simulink model "sim_sil_target_PWM_s32k1xx"  (Simulink 9.0)
settings: Solver=FixedStepDiscrete  StartTime=0.0  StopTime=12  FixedStep=1  RelTol=1e-3  EnableMultiTasking=on
InitFcn:
  | mbd_s32k_consistency_checks(bdroot(gcs));
undefined symbols (not defined in the file): LQFP
libraries: mbd_s32k1xx_ec_toolbox x2
settings Model: Creator=NXP MBDT Team  LastModifiedBy=nxf35172
settings DataIOCC: ExternalInput=off  InitialState=off  LimitDataPoints=on  SaveOutput=off  SignalLogging=off  SaveTime=off
settings OptimizationCC: DefaultParameterBehavior=Inlined  EnhancedBackFolding=on  PassReuseOutputArgsAs=Individual arguments  LifeSpan=auto  OptimizeBlockOrder=speed  DifferentSizesBufferReuse=on
settings DebuggingCC: UnderspecifiedInitializationDetection=Simplified  MergeDetectMultiDrivingBlocksExec=error  SolverPrmCheckMsg=warning  InheritedTsInSrcMsg=none  SingleTaskRateTransMsg=error  ParameterTunabilityLossMsg=error  UnconnectedInputMsg=error  UnconnectedOutputMsg=error  UnconnectedLineMsg=error  AllowSymbolicDim=off  UnknownTsInhSupMsg=error
settings HardwareCC: ProdIntDivRoundTo=Zero  ProdEndianess=LittleEndian  ProdHWDeviceType=Generic->Custom
settings SFSimCC: MATLABDynamicMemAlloc=off
settings RTWCC: SystemTargetFile=mbd_s32k.tlc  MakeCommand=mbd_s32k_make_rtw COPY_MDLREF_INCLUDES=0  TemplateMakefile=mbd_s32k.tmf  Description=Model Based Design Toolbox S32K1xx Code Generation Target  GenerateReport=on  IncludeHyperlinkInReport=on  LaunchReport=on  PortableWordSizes=on  GenerateTraceInfo=on  GenerateTraceReport=on  GenerateTraceReportSl=on  GenerateTraceReportSf=on  GenerateTraceReportEml=on
settings CodeAppCC: ForceParamTrailComments=on  IgnoreCustomStorageClasses=off  MaxIdLength=63  OperatorAnnotations=on  SimulinkDataObjDesc=on  SFDataObjDesc=on  InsertBlockDesc=on  StateflowObjectComments=off
settings STFCustomTargetCC: MultiwordLength=256  CombineOutputUpdateFcns=on  SuppressErrorStatus=on  ERTCustomFileBanners=on  SupportAbsoluteTime=off  SupportContinuousTime=off  SupportNonInlinedSFcns=off  RemoveResetFunc=on  MATLABClassNameForMDSCustomization=Simulink.SoftwareTarget.ERTCustomization  GRTInterface=off  SystemTargetFile=mbd_s32k.tlc
settings ERTTargetCC: ParMdlRefBuildCompliant=off  CompOptLevelCompliant=off  ConcurrentExecutionCompliant=off  SuppressErrorStatus=on  SupportAbsoluteTime=off  ModelStepFunctionPrototypeControlCompliant=off  CPPClassGenCompliant=off  UseToolchainInfoCompliant=off  InlinedParameterPlacement=NonHierarchical  ERTCustomFileTemplate=example_file_process.tlc

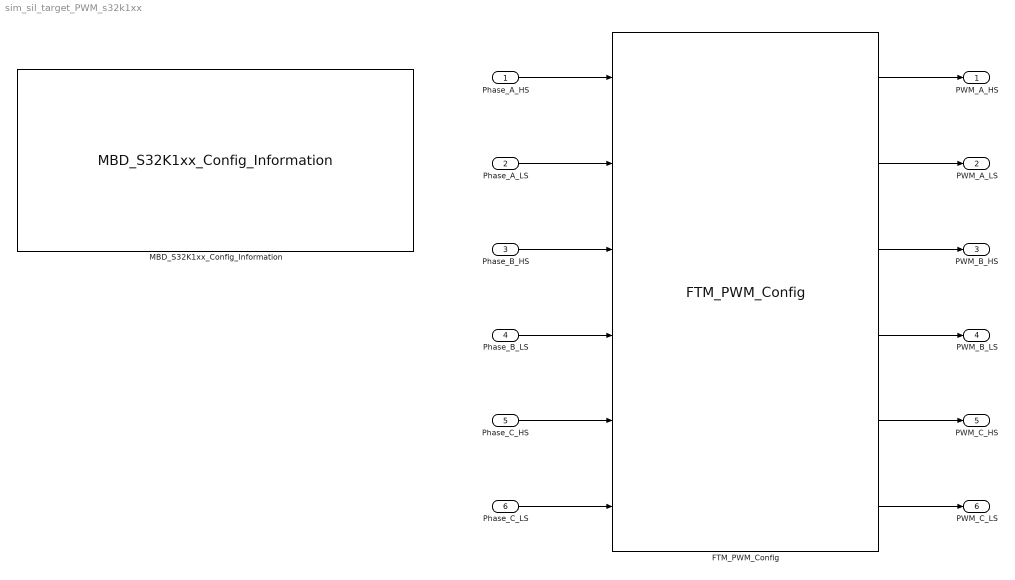
== system sim_sil_target_PWM_s32k1xx ==
  Phase_A_HS : Inport
  Phase_A_LS : Inport  Port=2
  Phase_B_HS : Inport  Port=3
  Phase_B_LS : Inport  Port=4
  Phase_C_HS : Inport  Port=5
  Phase_C_LS : Inport  Port=6
  FTM_PWM_Config : mbd_s32k1xx_ec_toolbox/Motor Control Blocks/FTM Blocks/FTM_PWM_Config  Priority=1  ftmModule=3  ftmMode=Center-Aligned PWM  ftmSourceClock=80 MHz  swcontrol_enable=off  chan0En=on  chan0Type=Independent  chan2En=on  chan2Type=Independent  chan4En=on  chan4Type=Independent  chan6En=off  chan6Type=Independent  ftmPwmUnits=Hz  outFrequency=1000  ftmPeriod=20000  ftmPrescaler=Divide by 4  deadtimeUnits=Nanoseconds  deadtimeNs=0  deadtimeTicks=0  deadtimePrescaler=Divide by 1  dutyCycleCh0=0.25  dutyCycleCh1=0.25  dutyCycleCh2=0.25  dutyCycleCh3=0.25  dutyCycleCh4=0.25  dutyCycleCh5=0.25  dutyCycleCh6=0.25  dutyCycleCh7=0.25  dutyCycleSim=on  startAfterInit=on  showAdvOpt=on  pinFtmCh0=PTB8: [FTM3_CH0 | FTM Channel]  pinFtmCh1=PTB9: [FTM3_CH1 | FTM Channel]  pinPolCh0=Active Low  pinPolCh1=Active Low  outputComplem0=Main duplicated  outputLevel0=Low  outputLevel1=Low  pinFtmCh2=PTB10: [FTM3_CH2 | FTM Channel]  pinFtmCh3=PTB11: [FTM3_CH3 | FTM Channel]  pinPolCh2=Active Low  pinPolCh3=Active Low  outputComplem2=Main duplicated  outputLevel2=Low  outputLevel3=Low  pinFtmCh4=PTC10: [FTM3_CH4 | FTM Channel]  pinFtmCh5=PTC11: [FTM3_CH5 | FTM Channel]  pinPolCh4=Active Low  pinPolCh5=Active Low  outputComplem4=Main duplicated  outputLevel4=Low  outputLevel5=Low  pinFtmCh6=PTC12: [FTM3_CH6 | FTM Channel]  pinFtmCh7=None  pinPolCh6=Active Low  pinPolCh7=Active Low  outputComplem6=Main duplicated  outputLevel6=Low  outputLevel7=Low  initTrigger=off  chTrigger0=off  chTrigger1=off  chTrigger2=off  chTrigger3=off  chTrigger4=off  chTrigger5=off  chTrigger6=off  chTrigger7=off  mcuTargetUpdate=on  pwmSyncTrg=Software trigger  pwmSyncHwRouting=TRGMUX_FTM7  pwmSyncTrg0=off  pwmSyncTrg1=off  pwmSyncTrg2=off  pwmSyncAutoClear=on  pwmSyncMinLoad=on  pwmSyncMaxLoad=on  pwmSyncInvert=System Clock  pwmSyncOutControl=System Clock  pwmSyncOutMask=System Clock  pwmSyncCounterInitial=System Clock  pwmSyncPoints=Update now  reloadEnable=off  reloadPriority=15  reloadHalfCycle=off  reloadHCR=0  reloadFrequency=0  chnMatch0=off  chnMatch1=off  chnMatch2=off  chnMatch3=off  chnMatch4=off  chnMatch5=off  chnMatch6=off  chnMatch7=off  pwmFaultProtection=off  pwmFaultInterrupt=off  pwmFaultClearing=Fault control disabled  pwmFaultPinState=Safe Value  pwmFaultFilterValue=0  pwmFaultPriority=15  fault_disen_0=off  fault_filter_0=off  fault_polarity_0=Active High  fault_disen_1=off  fault_filter_1=off  fault_polarity_1=Active high  fault_disen_2=off  fault_filter_2=off  fault_polarity_2=Active high  fault_disen_3=off  fault_filter_3=off  fault_polarity_3=Active high  fault_pin_0=None  fault_pin_1=None  fault_pin_2=None  fault_pin_3=None
  MBD_S32K1xx_Config_Information : mbd_s32k1xx_ec_toolbox/MBD_S32K1xx_Config_Information  mbdt_ver=0  disp_str=|  config_params=target_mcu::S32K144;;mcu_target_package::100-pin;;mcu_system_clock_freq::80;;mcu_xtal_freq::External 8;;mcu_systick_prio::15;;mcu_sys_tick_supress::off;;ds_import_enable::off;;target_compiler::GCC;;target_memory::FLASH;;gcc_target_compile_opts::-c -mcpu=cortex-m4 -mthumb -mfloat-abi=hard -mfpu=fpv4-sp-d16 -g -gstrict-dwarf;;gcc_target_assemble_opts::-mcpu=cortex-m4 -mfloat-abi=hard -mfpu=fpv4-sp-d16 -g;;gcc_target_link_opts::-mcpu=cortex-m4 -mthumb -mfloat-abi=hard -mfpu=fpv4-sp-d16;;gcc_target_lib_opts::;;gcc_target_default_lcf::on;;gcc_target_user_lcf::S32K144_100_flash.ld;;ghs_target_compile_opts::-cpu=cortexm4f -fpu=vfpv4_d16 -fsingle -mthumb -Wundef -Wimplicit-int -Wshadow -Wtrigraphs --no_commons --gnu_asm -gnu99 -O3 -Otime -gdwarf-2 -G ;;ghs_target_assemble_opts::-cpu=cortexm4f -fpu=vfpv4_d16;;ghs_target_link_opts::-cpu=cortexm4f -mthumb -fpu=vfpv4_d16;;ghs_target_lib_opts::;;ghs_target_default_lcf::on;;ghs_target_user_lcf::S32K144_100_flash.ld;;iar_target_compile_opts::--cpu=Cortex-M4F --fpu=VFPv4_sp -e --debug --dlib_config normal -Oh;;iar_target_assemble_opts::--cpu Cortex-M4F --fpu VFPv4_sp;;iar_target_link_opts::--no_exceptions --vfe --inline;;iar_target_lib_opts::;;iar_target_default_lcf::on;;iar_target_user_lcf::S32K144_100_flash.icf;;pil_download_enable::on;;rbl_download_enable::off;;rbl_restart_request::off;;rbl_start_delay::5000000;;rbl_com_port::1;;pil_download_rate::57600;;rbl_download_interface::OpenSDA;;pil_opensda_drive::E;;fmaster_enable::off;;fmaster_interface::UART0;;fmaster_uart_baud_rate::57600;;fmaster_uart0_rxd::PTA2 : [73] : [48] : [C10];;fmaster_uart0_txd::PTA3 : [72] : [47] : [D8];;fmaster_uart1_rxd::PTC6 : [81] : [52] : [C7];;fmaster_uart1_txd::PTC7 : [80] : [51] : [B8];;fmaster_uart2_rxd::PTD6 : [32] : [23] : [J4];;fmaster_uart2_txd::PTD7 : [31] : [22] : [K3];;fmaster_can0_rxd::PTE4 : [9] : [6] : [D1];;fmaster_can0_txd::PTE5 : [8] : [5] : [D2];;fmaster_can1_rxd::PTC6 : [81] : [52] : [C7];;fmaster_can1_txd::PTC7 : [80] : [51] : [B8];;fmaster_can2_rxd::PTC16 : [44] : [28] : [J7];;fmaster_can2_txd::PTC17 : [43] : [27] : [K7];;fmaster_can_baud_rate::1M;;ModelRef_PcrCheckEnDis::on;;ADC_PcrCheckEnDis::on;;AMMCLIB_PcrCheckEnDis::on;;CMP_PcrCheckEnDis::on;;FlexCAN_PcrCheckEnDis::on;;FM_pcrCheckEnDis::on;;FTM_Independent_Ouputs_PcrCheckEnDis::on;;FTM_Complementary_Ouputs_PcrCheckEnDis::on;;FTM_Three_Phase_Outputs_PcrCheckEnDis::on;;FTM_Input_Edge_Inputs_PcrCheckEnDis::on;;FTM_Dual_Edge_Inputs_PcrCheckEnDis::on;;FTM_Quadrature_Inputs_PcrCheckEnDis::on;;GPIO_OutputPcrCheckEnDis::on;;GPIO_InputPcrCheckEnDis::on;;LPI2C_PcrCheckEnDis::on;;LPSPI_PcrCheckEnDis::on;;LPUART_PcrCheckEnDis::on;;PDB0_PcrCheckEnDis::on;;PIT_PcrCheckEnDis::on;;Profile_PcrCheckEnDis::on;;  mcu_target_name=S32K144  mcu_target_package=100-LQFP  mcu_target_sram_size=48KB  mcu_system_clock_freq=80  mcu_xtal_freq=External 8  mcu_steptick_timer=LPIT Channel 0  mcu_steptick_prio=15  ds_import_enable=on  target_compiler=GCC  target_memory=FLASH  gcc_target_compile_opts=-mcpu=cortex-m4 -mthumb -mfloat-abi=hard -mfpu=fpv4-sp-d16 -O1 -g -gstrict-dwarf  gcc_target_assemble_opts=-mcpu=cortex-m4 -mthumb -mfloat-abi=hard -mfpu=fpv4-sp-d16 -g  gcc_target_link_opts=-mcpu=cortex-m4 -mthumb -mfloat-abi=hard -mfpu=fpv4-sp-d16  gcc_target_default_lcf=on  gcc_target_user_lcf=S32K144_48_flash.ld  ghs_target_compile_opts=-cpu=cortexm4f -thumb -DARM_MATH_CM4 -fpu=vfpv4_d16 -fsingle -Ogeneral -Wundef -Wimplicit-int -Wshadow -Wtrigraphs --no_commons --gnu_asm -gnu99 -gdwarf-2 -G  ghs_target_assemble_opts=-cpu=cortexm4f -fpu=vfpv4_d16  ghs_target_link_opts=-cpu=cortexm4f -thumb -fpu=vfpv4_d16  ghs_target_default_lcf=off  ghs_target_user_lcf=S32K144_48_flash.ld  iar_target_compile_opts=--cpu=Cortex-M4F --thumb --fpu=VFPv4_sp -Ol -e --debug --dlib_config normal  iar_target_assemble_opts=--cpu Cortex-M4F --thumb --fpu VFPv4_sp  iar_target_link_opts=--no_exceptions --vfe --inline  iar_target_default_lcf=off  iar_target_user_lcf=S32K144_48_flash.icf  pil_download_enable=off  rbl_download_enable=off  rbl_start_delay=5000000  rbl_download_interface=OpenSDA  rbl_restart_request=off  rbl_com_port=Custom  rbl_com_port_custom=COM1  pil_download_rate=57600  pil_opensda_drive=Custom  pil_opensda_drive_custom=D  pil_uart_instance=0  pil_uart_rx=PTA2: [LPUART0_RX | Receive]  pil_uart_tx=PTA3: [LPUART0_TX | Transmit]  FTM_PWM_PcrCheckEnDis=on  FTM_Input_Edge_Inputs_PcrCheckEnDis=on  FTM_Dual_Edge_Inputs_PcrCheckEnDis=on  FTM_Quadrature_Inputs_PcrCheckEnDis=on  FTM_Hall_Sensor_Inputs_PcrCheckEnDis=on  LPTMR_PcrCheckEnDis=on  PIT_PcrCheckEnDis=on  RTC_PcrCheckEnDis=on  FlexCAN_PcrCheckEnDis=on  LIN_PcrCheckEnDis=on  FlexIO_PcrCheckEnDis=on  LPI2C_PcrCheckEnDis=on  LPSPI_PcrCheckEnDis=on  LPUART_PcrCheckEnDis=on  CMP_PcrCheckEnDis=on  GPIO_OutputPcrCheckEnDis=on  GPIO_InputPcrCheckEnDis=on  SBC_PcrCheckEnDis=on  AMMCLIB_PcrCheckEnDis=on  FM_PcrCheckEnDis=on  Profile_PcrCheckEnDis=on  ConfigParams_PcrCheckEnDis=on  ModelRef_PcrCheckEnDis=on  PDB0_PcrCheckEnDis=on  CSEc_PcrCheckEnDis=on  eDMA_PcrCheckEnDis=on  ADC_PcrCheckEnDis=on  WDOG_PcrCheckEnDis=on
      | Target : S32K144
      | Package : 100-pin
      | System clock : 80 MHz
      | XTAL clock : External 8 MHz
      | Compiler : GCC
      | Target Type : FLASH
      | Processor-In-Loop : (COM1, 57600, OpenSDA: E)
      | Freemaster : None
      | System Tick Interrupt Priority : 15
  PWM_A_HS : Outport
  PWM_A_LS : Outport  Port=2
  PWM_B_HS : Outport  Port=3
  PWM_B_LS : Outport  Port=4
  PWM_C_HS : Outport  Port=5
  PWM_C_LS : Outport  Port=6
  wires:
  Phase_A_HS/1 -> FTM_PWM_Config/1
  Phase_A_LS/1 -> FTM_PWM_Config/2
  Phase_B_HS/1 -> FTM_PWM_Config/3
  Phase_B_LS/1 -> FTM_PWM_Config/4
  Phase_C_HS/1 -> FTM_PWM_Config/5
  Phase_C_LS/1 -> FTM_PWM_Config/6
  FTM_PWM_Config/1 -> PWM_A_HS/1
  FTM_PWM_Config/2 -> PWM_A_LS/1
  FTM_PWM_Config/3 -> PWM_B_HS/1
  FTM_PWM_Config/4 -> PWM_B_LS/1
  FTM_PWM_Config/5 -> PWM_C_HS/1
  FTM_PWM_Config/6 -> PWM_C_LS/1
